simulink model "design_optimization"  (R2024b)
settings: Solver=FixedStepAuto  StartTime=0.0  StopTime=100  FixedStep=0.01  RelTol=1e-3
model workspace (MAT data in the model file):
  Kd = 11.2358411832
  Ki = 0.257144197246
  Kp = 0.507737893263
  design_optimization_sdosession = sldodialogs.data.SessionData
  design_optimization_sdosession.Version = '4.0'
  design_optimization_sdosession.Data.ModelName = 'design_optimization'
  design_optimization_sdosession.Data.ToolType = 'ResponseOptimization'
  design_optimization_sdosession.Data.GUIOptions.NoPromptClose = 0
  design_optimization_sdosession.Data.Workspace.LocalWorkspace.BlockReq = sldodialogs.databrowser.BlockRequirementData
  design_optimization_sdosession.Data.Workspace.LocalWorkspace.BlockReq.Name = 'BlockReq'
  design_optimization_sdosession.Data.Workspace.LocalWorkspace.BlockReq.Block = 'design_optimization/Check Step Response 
    | Characteristics'
  design_optimization_sdosession.Data.Workspace.LocalWorkspace.DesignVars(1) = param.Continuous
  design_optimization_sdosession.Data.Workspace.LocalWorkspace.DesignVars(1).Minimum_ = 0.001
  design_optimization_sdosession.Data.Workspace.LocalWorkspace.DesignVars(1).Scale_ = 16
  design_optimization_sdosession.Data.Workspace.LocalWorkspace.DesignVars(1).Size_ = [1 1]
  design_optimization_sdosession.Data.Workspace.LocalWorkspace.DesignVars(1).Value_ = 11.2358411832
  design_optimization_sdosession.Data.Workspace.LocalWorkspace.DesignVars(1).pID = paramid.Variable
  design_optimization_sdosession.Data.Workspace.LocalWorkspace.DesignVars(1).pID.Name = 'Kd'
  design_optimization_sdosession.Data.Workspace.LocalWorkspace.DesignVars(2) = param.Continuous
  design_optimization_sdosession.Data.Workspace.LocalWorkspace.DesignVars(2).Minimum_ = 0.001
  design_optimization_sdosession.Data.Workspace.LocalWorkspace.DesignVars(2).Scale_ = 0.5
  design_optimization_sdosession.Data.Workspace.LocalWorkspace.DesignVars(2).Size_ = [1 1]
  design_optimization_sdosession.Data.Workspace.LocalWorkspace.DesignVars(2).Value_ = 0.257144197246
  design_optimization_sdosession.Data.Workspace.LocalWorkspace.DesignVars(2).pID = paramid.Variable
  design_optimization_sdosession.Data.Workspace.LocalWorkspace.DesignVars(2).pID.Name = 'Ki'
  design_optimization_sdosession.Data.Workspace.LocalWorkspace.DesignVars(3) = param.Continuous
  design_optimization_sdosession.Data.Workspace.LocalWorkspace.DesignVars(3).Minimum_ = 0.001
  design_optimization_sdosession.Data.Workspace.LocalWorkspace.DesignVars(3).Size_ = [1 1]
  design_optimization_sdosession.Data.Workspace.LocalWorkspace.DesignVars(3).Value_ = 0.507737893263
  design_optimization_sdosession.Data.Workspace.LocalWorkspace.DesignVars(3).pID = paramid.Variable
  design_optimization_sdosession.Data.Workspace.LocalWorkspace.DesignVars(3).pID.Name = 'Kp'
  design_optimization_sdosession.Data.Workspace.LocalWorkspace.ReqValues.Name = 'design_optimization/Check Step Response 
    | Characteristics (Upper)'
  design_optimization_sdosession.Data.Workspace.LocalWorkspace.ReqValues.Type = '<='
  design_optimization_sdosession.Data.Workspace.LocalWorkspace.ReqValues.Value = [-1.33136204742e-05; -0.000265176898474; -0.00368255564461; 0; -0.258713997001; -0.00691193383191; -0.000162399517626; -0.528682975073]
  design_optimization_sdosession.Data.Workspace.LocalWorkspace.ReqValues.DisplayValue = [-1.33136204742e-05; -0.000265176898474; -0.00368255564461; 0; -0.258713997001; -0.00691193383191; -0.000162399517626; -0.528682975073]
  design_optimization_sdosession.Data.Workspace.HiddenWorkspace = []
  design_optimization_sdosession.Data.ToolData.DialogManager = []
  design_optimization_sdosession.Data.ToolData.PlotManager.Plots.Class = 'block'
  design_optimization_sdosession.Data.ToolData.PlotManager.Plots.Sources{1} = 'design_optimization/Check Step Response 
    | Characteristics'
  design_optimization_sdosession.Data.ToolData.PlotManager.Tiling.gridDimensions.w = 1
  design_optimization_sdosession.Data.ToolData.PlotManager.Tiling.gridDimensions.h = 1
  design_optimization_sdosession.Data.ToolData.PlotManager.Tiling.tileCount = 1
  design_optimization_sdosession.Data.ToolData.PlotManager.Tiling.tileCoverage = 1
  design_optimization_sdosession.Data.ToolData.PlotManager.Tiling.referenceWidth = 824
  design_optimization_sdosession.Data.ToolData.PlotManager.Tiling.referenceHeight = 456
  design_optimization_sdosession.Data.ToolData.PlotManager.Tiling.columnWeights = 1
  design_optimization_sdosession.Data.ToolData.PlotManager.Tiling.rowWeights = 1
  design_optimization_sdosession.Data.ToolData.PlotManager.Tiling.columnLeft = [0; 824]
  design_optimization_sdosession.Data.ToolData.PlotManager.Tiling.rowTop = [0; 456]
  design_optimization_sdosession.Data.ToolData.PlotManager.Tiling.tileOccupancy.children.showOrder = 0
  design_optimization_sdosession.Data.ToolData.PlotManager.Tiling.tileOccupancy.children.id = 'PlotManager 3679504f-166f-47df-87d0-47c340bfb27b_TimePlot aaa5dce3-b7a9-4843-b75f-424f0f7aa016'
  design_optimization_sdosession.Data.ToolData.PlotManager.Tiling.tileOccupancy.children.title = 'Time plot 1'
  design_optimization_sdosession.Data.ToolData.PlotManager.Tiling.tileOccupancy.showingChildId = 'PlotManager 3679504f-166f-47df-87d0-47c340bfb27b_TimePlot aaa5dce3-b7a9-4843-b75f-424f0f7aa016'
  design_optimization_sdosession.Data.ToolData.PlotManager.Tiling.tileOccupancy.showingChildTitle = 'Time plot 1'
  design_optimization_sdosession.Data.ToolData.PlotManager.Tiling.emptyTileCount = 0
  design_optimization_sdosession.Data.ToolData.PlotManager.Tiling.selectionOrder.PlotManager3679504f_166f_47df_87d0_47c340bfb27b_TimePlotAaa5dce = 1
  design_optimization_sdosession.Data.ToolData.ResponseOptimization.Options = sdo.OptimizeOptions
  design_optimization_sdosession.Data.ToolData.ResponseOptimization.Options.OptimizedModel = 'design_optimization'
  design_optimization_sdosession.Data.ToolData.ResponseOptimization.Options.Version = 2
  design_optimization_sdosession.Data.ToolData.ResponseOptimization.GUIOptions.ModelTimeOut = Inf
  design_optimization_sdosession.Data.ToolData.ResponseOptimization.GUIOptions.ComputeOperatingPoint = 0
  design_optimization_sdosession.Data.ToolData.ResponseOptimization.GUIOptions.ShowProgress = 1
  design_optimization_sdosession.Data.ToolData.ResponseOptimization.GUIOptions.ShowParamTrajectory = 1
  design_optimization_sdosession.Data.ToolData.ResponseOptimization.GUIOptions.UpdatePlots = 1
  design_optimization_sdosession.Data.ToolData.ResponseOptimization.GUIOptions.UpdateModel = 1
  design_optimization_sdosession.Data.ToolData.ResponseOptimization.GUIOptions.UpdateDesign = 'overwrite'
  design_optimization_sdosession.Data.ToolData.ResponseOptimization.GUIOptions.SaveReport = 0
  design_optimization_sdosession.Data.ToolData.ResponseOptimization.GUIOptions.SaveRequirementValue = 1
  design_optimization_sdosession.Data.ToolData.ResponseOptimization.LinOptions = linearize.LinearizeOptions
  design_optimization_sdosession.Data.ToolData.ResponseOptimization.RequirementOperatingPointSetup = []
  design_optimization_sdosession.Data.ToolData.ResponseOptimization.LocalRequirements = struct([])
  design_optimization_sdosession.Data.ToolData.ResponseOptimization.BlockRequirements.Block = 'design_optimization/Check Step Response 
    | Characteristics'
  design_optimization_sdosession.Data.ToolData.ResponseOptimization.BlockRequirements.Selected = 1
  design_optimization_sdosession.Data.ToolData.ResponseOptimization.BlockRequirements.hReq = sdo.requirements.StepResponseEnvelope
  design_optimization_sdosession.Data.ToolData.ResponseOptimization.BlockRequirements.hReq.sdo.requirements.Requirement.Data_ = srorequirement.steprespdata
  design_optimization_sdosession.Data.ToolData.ResponseOptimization.BlockRequirements.hReq.sdo.requirements.Requirement.Data_.Linked = [0  0; 0  0; 0  0; 0  0]
  design_optimization_sdosession.Data.ToolData.ResponseOptimization.BlockRequirements.hReq.sdo.requirements.Requirement.Data_.OpenEnd = [0; 1]
  design_optimization_sdosession.Data.ToolData.ResponseOptimization.BlockRequirements.hReq.sdo.requirements.Requirement.Data_.Weight = [1; 1; 1; 1; 1]
  design_optimization_sdosession.Data.ToolData.ResponseOptimization.BlockRequirements.hReq.sdo.requirements.Requirement.Data_.xCoords = [0  15; 15  22.5; 0  5; 5  15; 15  22.5]
  design_optimization_sdosession.Data.ToolData.ResponseOptimization.BlockRequirements.hReq.sdo.requirements.Requirement.Data_.xUnits = 'seconds'
  design_optimization_sdosession.Data.ToolData.ResponseOptimization.BlockRequirements.hReq.sdo.requirements.Requirement.Data_.yCoords = [1.1  1.1; 1.01  1.01; 0  0; 0.8  0.8; 0.99  0.99]
  design_optimization_sdosession.Data.ToolData.ResponseOptimization.BlockRequirements.hReq.sdo.requirements.Requirement.Check_ = sdo.requirements.PiecewiseLinearCheck
  design_optimization_sdosession.Data.ToolData.ResponseOptimization.BlockRequirements.hReq.sdo.requirements.Requirement.Check_.Orientation = 'horizontal'
  design_optimization_sdosession.Data.ToolData.ResponseOptimization.BlockRequirements.hReq.sdo.requirements.Requirement.Check_.XScale = 'linear'
  design_optimization_sdosession.Data.ToolData.ResponseOptimization.LocalExperiments = struct([])
  design_optimization_sdosession.Data.ToolData.ResponseOptimization.Cost.Type = 'SSE'
  design_optimization_sdosession.Data.ToolData.ResponseOptimization.Cost.Robust = 'off'
  design_optimization_sdosession.Data.ToolData.ResponseOptimization.DesignVariables = 'DesignVars'
  design_optimization_sdosession.Data.ToolData.ResponseOptimization.UncertainVariables = ''
  design_optimization_sdosession.Data.ToolData.ResponseOptimization.DataToPlot = ''
libraries: checkpacklib x1, slpidlib x1
settings Model: Creator=arthu  LastModifiedBy=arthu

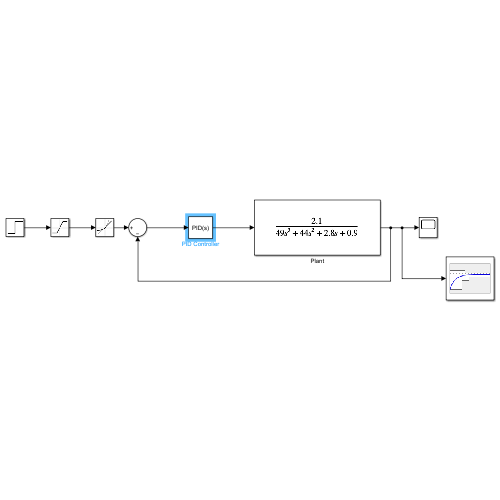
[thumbnail: Simulink's stored preview of the top-level diagram]
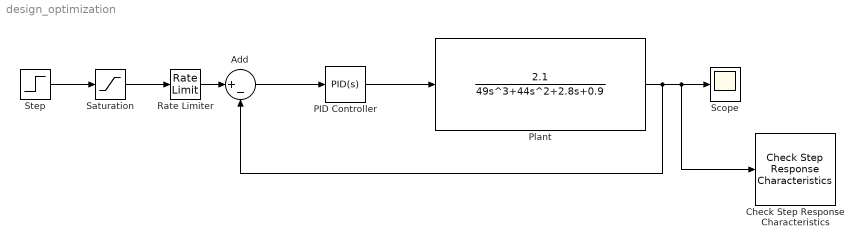
== system design_optimization ==
  Add : Sum  Inputs=|+-
  Check Step Response Characteristics : checkpacklib/Check Step Response  Characteristics  InstantiateOnLoad=on  enabled=on  stopWhenAssertionFail=off  export=off  ViewDlgPos=[100 200 510 390]  OpenViewOnLoad=off  LaunchViewOnOpen=off  TimeUnits=seconds  EnableStepResponseBound=on  InitialValue=0  FinalValue=1  StepTime=0  RiseTime=5  PercentRise=80  SettlingTime=15  PercentSettling=1  PercentOvershoot=10  PercentUndershoot=0
      settings: LibrarySourceBlock=|
      | sdolib/Model Verification/Check Step Response
      | Characteristics
  PID Controller : slpidlib/PID Controller  Controller=PID  Form=Parallel  TimeDomain=Continuous-time  UseExternalTs=off  SampleTime=-1  IntegratorMethod=Forward Euler  FilterMethod=Forward Euler  ControllerParametersSource=internal  P=Kp  I=Ki  UseKiTs=off  D=Kd  UseExternalDerivativeSource=off  N=100  UseFilter=on  TunerSelectOption=Transfer Function Based (PID Tuner App)  InitialConditionSource=internal  InitialConditionForIntegrator=0  InitialConditionForFilter=0  DifferentiatorICPrevScaledInput=0  ExternalReset=none  TrackingMode=off  Kt=1  LimitOutput=off  SatLimitsSource=internal  UpperSaturationLimit=inf  LowerSaturationLimit=-inf  LinearizeAsGain=on  AntiWindupMode=none  Kb=1  LimitIntegrator=off  UpperIntegratorSaturationLimit=inf  LowerIntegratorSaturationLimit=-inf  POutMin=[]  POutMax=[]  IOutMin=[]  IOutMax=[]  DOutMin=[]  DOutMax=[]  NOutMin=[]  NOutMax=[]  SumOutMin=[]  SumOutMax=[]  SaturationOutMin=[]  SaturationOutMax=[]  PParamMin=[]  PParamMax=[]  IParamMin=[]  IParamMax=[]  DParamMin=[]  DParamMax=[]  NParamMin=[]  NParamMax=[]  KbParamMin=[]  KbParamMax=[]  KtParamMin=[]  KtParamMax=[]  KbOutMin=[]  KbOutMax=[]  KtOutMin=[]  KtOutMax=[]  IntegratorOutMin=[]  IntegratorOutMax=[]  FilterOutMin=[]  FilterOutMax=[]  SumI1OutMin=[]  SumI1OutMax=[]  SumI2OutMin=[]  SumI2OutMax=[]  SumI3OutMin=[]  SumI3OutMax=[]  SumI4OutMin=[]  SumI4OutMax=[]  SumDOutMin=[]  SumDOutMax=[]  DifferentiatorOutMin=[]  DifferentiatorOutMax=[]  FilterDiffOutCoefMin=[]  FilterDiffOutCoefMax=[]  ReciprocalOutMin=[]  ReciprocalOutMax=[]  SumDenOutMin=[]  SumDenOutMax=[]  SumNumOutMin=[]  SumNumOutMax=[]  DivideOutMin=[]  DivideOutMax=[]  UdiffTsProdOutMin=[]  UdiffTsProdOutMax=[]  NTsProdOutMin=[]  NTsProdOutMax=[]  UintegralTsProdOutMin=[]  UintegralTsProdOutMax=[]  UngainTsProdOutMin=[]  UngainTsProdOutMax=[]  ClampingZeroOutDataTypeStr=Inherit: Inherit via back propagation  ClampingZeroOutMin=[]  ClampingZeroOutMax=[]  FilterDenConstantOutDataTypeStr=Inherit: Inherit via back propagation  FilterDenConstantOutMin=[]  FilterDenConstantOutMax=[]  PCopyOutDataTypeStr=Inherit: Inherit via back propagation  PCopyOutMin=[]  PCopyOutMax=[]  NCopyOutDataTypeStr=Inherit: Inherit via back propagation  NCopyOutMin=[]  NCopyOutMax=[]  IntegratorContinuousStateAttributes=''  IntegratorStateMustResolveToSignalObject=off  IntegratorRTWStateStorageClass=Auto  FilterContinuousStateAttributes=''  FilterStateMustResolveToSignalObject=off  FilterRTWStateStorageClass=Auto  ParallelPVariant=InternalParameters  IdealPVariant=Disabled  IVariant=InternalParameters  DVariant=InternalParameters  IntegratorVariant=Continuous  SatVariant=Disabled  AWVariant=Passthrough  PCopyVariant=Disabled  TRVariant=Disabled  FdbkBlocksVariant=Forward  IdealPFdbkVariant=Disabled  SatFdbkVariant=Disabled  DerivativeFilterVariant=ContFilter  NVariant=InternalParameters  NCopyVariant=Disabled  FilterICVariant=InternalICsFilter  IntegratorICVariant=InternalICs  ExternalResetVariant=Disabled  TRSumVariant=Passthrough  SumFdbkVariant=Disabled  SumVariant=Sum_PID  TsampFilterVariant=InternalTs  TsampNgainVariant=Passthrough  TsampIntegralVariant=Disabled_SignalSpec  ExternalSaturationOutDataTypeStr=Inherit: Same as second input  DerivativeSourceVariant=ErrorSignal  PreIntVariant=InternalPreInt
  Plant : TransferFcn  Numerator=[2.1]  Denominator=[49 44 2.8 0.9]
  Rate Limiter : RateLimiter  RisingSlewLimit=0.8  FallingSlewLimit=-0.8  SampleTimeMode=inherited
  Saturation : Saturate  UpperLimit=2  LowerLimit=-2
  Scope : Scope
  Step : Step  Time=0  SampleTime=0
  wires:
  Step/1 -> Saturation/1
  Saturation/1 -> Rate Limiter/1
  PID Controller/1 -> Plant/1
  Plant/1 -> Check Step Response Characteristics/1, Scope/1, Add/2
  Rate Limiter/1 -> Add/1
  Add/1 -> PID Controller/1
